simulink model "SMC_asintotico"  (R2026b)
settings: Solver=ode4  StopTime=20  FixedStep=0.0001
settings Model: Creator=nestorhernandezcastellanos  LastModifiedBy=nestorhernandezcastellanos

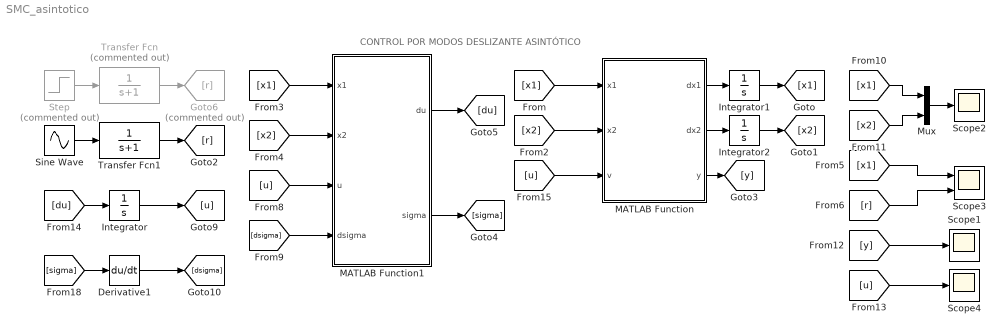
== system SMC_asintotico ==
  note: CONTROL POR MODOS DESLIZANTE ASINTÓTICO
  Derivative1 : Derivative
  Goto6 : Goto  Commented=on  GotoTag=r
  Integrator : Integrator
  Integrator1 : Integrator  InitialCondition=1
  Integrator2 : Integrator  InitialCondition=-2
  MATLAB Function : MATLAB Function  TreatAsAtomicUnit=on
  MATLAB Function1 : MATLAB Function  TreatAsAtomicUnit=on
  Mux : Mux  Inputs=2
  Scope1 : Scope
      settings: ActiveDisplayYMinimum=-1.1345018827917306  ActiveDisplayYMaximum=0.21051694512557476
  Scope2 : Scope
      settings: ActiveDisplayYMinimum=-2.4062422690892262  ActiveDisplayYMaximum=1.3784713632321361  DataLoggingVariableName=ScopeData2
  Scope3 : Scope  NumInputPorts=2
      settings: ActiveDisplayYMinimum=-0.92049512009098344  ActiveDisplayYMaximum=1.2133883466767759  DataLoggingVariableName=ScopeData3
  Scope4 : Scope
      settings: ActiveDisplayYMinimum=-26.249333606618752  ActiveDisplayYMaximum=26.244002459568783
  Sine Wave : Sin  SampleTime=0
  Step : Step  Commented=on  Time=10  SampleTime=0
  Transfer Fcn : TransferFcn  Commented=on  Denominator=[1 1]
  Transfer Fcn1 : TransferFcn  Denominator=[1 1]
  wires:
  MATLAB Function1/1(du) -> [du]
  MATLAB Function/2(dx2) -> Integrator2/1
  MATLAB Function/1(dx1) -> Integrator1/1
  Mux/1 -> Scope2/1
  Sine Wave/1 -> Transfer Fcn1/1
  [x1] -> MATLAB Function/1(x1)
  [x2] -> MATLAB Function/2(x2)
  [x1] -> MATLAB Function1/1(x1)
  [x2] -> MATLAB Function1/2(x2)
  [x1] -> Scope3/1
  [r] -> Scope3/2
  Integrator2/1 -> [x2]
  Integrator1/1 -> [x1]
  MATLAB Function/3(y) -> [y]
  [x2] -> Mux/2
  [x1] -> Mux/1
  [y] -> Scope1/1
  [u] -> Scope4/1
  Step/1 -> Transfer Fcn/1
  Derivative1/1 -> [dsigma]
  [sigma] -> Derivative1/1
  Integrator/1 -> [u]
  [du] -> Integrator/1
  [u] -> MATLAB Function1/3(u)
  [dsigma] -> MATLAB Function1/4(dsigma)
  MATLAB Function1/2(sigma) -> [sigma]
  [u] -> MATLAB Function/3(v)
  Transfer Fcn/1 -> Goto6/1
  Transfer Fcn1/1 -> [r]

== matlab function SMC_asintotico/MATLAB Function1 ==
  data: x1 input; x2 input; u input; du output; dsigma input; sigma output
function [du, sigma]= controlador(x1, x2, u, dsigma)

% Ganancia K>1
K = 10;

% Valor arbitrario positivo
m = 4;
ms = 5;

sigma = x2 + m*x1;
s = dsigma + ms*sigma;
du = -m*ms*x2 - (m+ms)*u - K*sign(s);

== matlab function SMC_asintotico/MATLAB Function ==
  data: x1 input; x2 input; dx1 output; v input; dx2 output; y output
function [dx1, dx2, y] = planta(x1, x2, v)

dx1 = x2;
dx2 = sin(x1+x2) + cos(x1*x2) + v;

y = x1;
